simulink subsystem "PowerSystemRef"  (R2024b)
settings: Solver=VariableStepAuto  StartTime=0.0  StopTime=10.0  RelTol=1e-3
undefined symbols (not defined in the file): ess, geom, mot, mot2, mot3, mot4, propel, propel2, propel3, propel4, pxf_diagram_options, SimIn, tc, tc2, tc3, tc4
libraries: simulink x10, slpidlib x5
(part 8 of 10)

== system PowerSystemRef/powerplant/mot3/ctrl/dmd/parameter_selection ==
  inport-main_info_bus-1 : Inport
  select_main_info_bus : BusSelector  OutputSignals=apc_info_bus.apc_ctrl_dt3_simu,env_info_bus.env_plant_density_simu,apa_info_bus.powerplant_info_bus.ess.ctrl.ess_ctrl_pwr_max_pro_simu,apa_info_bus.powerplant_info_bus.propel3.propel3_plant_speed_simu,apa_info_bus.powerplant_info_bus.tc3.tc3_plant_spd_in_simu
  outport-apc_ctrl_dt3_simu-1 : Outport
  outport-env_plant_density_simu-2 : Outport  Port=2
  outport-ess_ctrl_pwr_max_pro_simu-3 : Outport  Port=3
  outport-propel3_plant_speed_simu-4 : Outport  Port=4
  outport-tc3_plant_spd_in_simu-5 : Outport  Port=5
  wires:
  inport-main_info_bus-1/1 -> select_main_info_bus/1
  select_main_info_bus/1 -> outport-apc_ctrl_dt3_simu-1/1  "<apc_ctrl_dt3_simu>"
  select_main_info_bus/2 -> outport-env_plant_density_simu-2/1  "<env_plant_density_simu>"
  select_main_info_bus/3 -> outport-ess_ctrl_pwr_max_pro_simu-3/1  "<ess_ctrl_pwr_max_pro_simu>"
  select_main_info_bus/4 -> outport-propel3_plant_speed_simu-4/1  "<propel3_plant_speed_simu>"
  select_main_info_bus/5 -> outport-tc3_plant_spd_in_simu-5/1  "<tc3_plant_spd_in_simu>"

== system PowerSystemRef/powerplant/mot3/plant/mot3_plant_map_Pelec_funTW_volt_in/electric machine filter ==
  trq : Inport
  Interval Test : simulink/Logic and Bit Operations/Interval Test  IntervalClosedRight=on  uplimit=0.02  IntervalClosedLeft=on  lowlimit=-0.02  OutDataTypeStr=boolean
  Switch : Switch  Threshold=0.5  SaturateOnIntegerOverflow=off  InputSameDT=off
  electric machine time response : TransferFcn  Denominator=[mot3.plant.init.time_response 1]
  filtered : Outport
  wires:
  Switch/1 -> filtered/1
  trq/1 -> electric machine time response/1, Interval Test/1, Switch/1
  Interval Test/1 -> Switch/2
  electric machine time response/1 -> Switch/3

== system PowerSystemRef/powerplant/mot3/plant/mot3_plant_map_Pelec_funTW_volt_in/max torque  ==
  cmd : Inport
  speed : Inport  Port=2
  torque : Inport  Port=3
  Abs : Abs
  Cont trq max - Prop : Subsystem  mask{x=mot3.plant.init.trq_pos_cont.idx1_spd, map=mot3.plant.init.trq_pos_cont.map}
      mask Display: image(imread('map1D.jpg','jpeg'))
  Cont trq max - Regen : Subsystem  mask{x=mot3.plant.init.trq_neg_cont.idx1_spd, map=mot3.plant.init.trq_neg_cont.map}
      mask Display: image(imread('map1D.jpg','jpeg'))
  Heat index : Subsystem
  Memory : Memory
  Peak trq max - Prop : Subsystem  mask{x=mot3.plant.init.trq_pos_max.idx1_spd, map=mot3.plant.init.trq_pos_max.map}
      mask Display: image(imread('map1D.jpg','jpeg'))
  Peak trq max - Regen : Subsystem  mask{x=mot3.plant.init.trq_neg_max.idx1_spd, map=mot3.plant.init.trq_neg_max.map}
      mask Display: image(imread('map1D.jpg','jpeg'))
  Product2 : Product  InputSameDT=on  SaturateOnIntegerOverflow=on  OutDataTypeStr=Inherit: Same as first input
  Product3 : Product  InputSameDT=on  SaturateOnIntegerOverflow=on  OutDataTypeStr=Inherit: Same as first input
  Product5 : Product  InputSameDT=on  SaturateOnIntegerOverflow=on  OutDataTypeStr=Inherit: Same as first input
  Sign : Signum
  Sum : Sum  InputSameDT=on  SaturateOnIntegerOverflow=on  OutDataTypeStr=Inherit: Same as first input
  Sum1 : Sum  Inputs=-+  InputSameDT=on  SaturateOnIntegerOverflow=on  OutDataTypeStr=Inherit: Same as first input
  Switch : Switch  InputSameDT=off
  Switch1 : Switch  InputSameDT=off
  cst : Constant
  max torque : Outport
  heat index : Outport  Port=2
  wires:
  Memory/1 -> Cont trq max - Prop/1(input x), Cont trq max - Regen/1(input x), Peak trq max - Regen/1(input x), Peak trq max - Prop/1(input x)
  Sign/1 -> Product5/1
  Product5/1 -> max torque/1
  Sum/1 -> Sign/1, Abs/1
  Abs/1 -> Product5/2
  torque/1 -> Heat index/2(torque)
  cmd/1 -> Switch1/2, Switch/2
  speed/1 -> Memory/1
  Cont trq max - Prop/1(output) -> Switch/1
  Cont trq max - Regen/1(output) -> Switch/3
  Peak trq max - Prop/1(output) -> Switch1/1
  Peak trq max - Regen/1(output) -> Switch1/3
  Switch/1 -> Product2/1, Heat index/1(cont torque)
  Switch1/1 -> Product3/2
  Product2/1 -> Sum/1
  Sum1/1 -> Product3/1
  Product3/1 -> Sum/2
  cst/1 -> Sum1/2
  Heat index/1(Heat index) -> Product2/2, Sum1/1, heat index/1

== system PowerSystemRef/powerplant/mot3/plant/mot3_plant_map_Pelec_funTW_volt_in/non-zero division ==
  note: and finally, the expression is: (u[1] \ u[2]) * 1 = u[1] \ u[2]
  note: (u[2]!=0) is true then returns 1
  note: if u[2] != 0, then output == u[1]\u[2]:
  note: (u[2]==0) is false then returns 0, thus (u[2]+(u[2]==0)) is equal to u[2]+0=u[2]
  note: and finally, the expression is: (u[1] \ 1) * 0 = 0
  note: (u[2]!=0) is false then returns 0
  note: if u[2] == 0, then output == 0:
  note: (u[2]==0) is true then returns 1, thus (u[2]+(u[2]==0)) is equal to 0+1=1
  note: original idea from Phil Sharer - ANL
      | original formula: u[1]\(u[2]+eps)*(u[2]!=0)
      | changes done by Gerald ZINI (dgey) - ANL (05\02\2001)
  In1 : Inport
  In2 : Inport  Port=2
  Fcn : Fcn  Expr=u[1]/(u[2]+(u[2]==0))*(u[2]!=0)
  Mux : Mux  Inputs=2
  Out1 : Outport
  wires:
  In2/1 -> Mux/2
  Fcn/1 -> Out1/1
  In1/1 -> Mux/1
  Mux/1 -> Fcn/1

== system PowerSystemRef/powerplant/mot4/ctrl/cmd/mot4_ctrl_cmd_map_Pelec_funTW_volt_in ==
  mot_plant_spd_out_simu : Inport
  mot_ctrl_trs_trq_simu : Inport  Port=2
  mot_ctrl_cstr_trq_max_pos_simu : Inport  Port=3
  mot_ctrl_cstr_trq_max_neg_simu : Inport  Port=4
  Abs : Abs
  Abs1 : Abs
  Abs2 : Abs
  Fcn : Fcn  Expr=(u>=0) - (u<0)
  Product : Product  SaturateOnIntegerOverflow=on  OutDataTypeStr=Inherit: Same as first input
  Product1 : Product  SaturateOnIntegerOverflow=on  OutDataTypeStr=Inherit: Same as first input
  Subsystem2 : Subsystem
      mask Display: disp('divider')
  Switch : Switch  InputSameDT=off
  "[-1, 1]" : Saturate  UpperLimit=1  LowerLimit=-1
  avoid zero output : Subsystem
  mot_ctrl_cmd_simu : Outport
  wires:
  avoid zero output/1(Out1) -> Product/2
  [mot4_ctrl_cmd_simu] -> mot_ctrl_cmd_simu/1  "mot_ctrl_cmd_simu"
  Product1/1 -> [mot4_ctrl_cmd_simu]
  mot_ctrl_cstr_trq_max_pos_simu/1 -> Abs1/1
  mot_ctrl_cstr_trq_max_neg_simu/1 -> Abs2/1
  mot_plant_spd_out_simu/1 -> avoid zero output/1(In1)
  Product/1 -> Switch/2, Fcn/1
  Switch/1 -> Subsystem2/2(In2)
  Subsystem2/1(Out1) -> "[-1, 1]"/1
  mot_ctrl_trs_trq_simu/1 -> Product/1, Abs/1
  Abs/1 -> Subsystem2/1(In1)
  Abs1/1 -> Switch/1
  Abs2/1 -> Switch/3
  "[-1, 1]"/1 -> Product1/2
  Fcn/1 -> Product1/1

== system PowerSystemRef/powerplant/mot4/ctrl/cmd/parameter_out ==
  inport-mot4_ctrl_cmd_simu : Inport
  Toworkspace-mot4_ctrl_cmd_simu : ToWorkspace  VariableName=mot4_ctrl_cmd_simu  SampleTime=pxf_diagram_options.workspace_sample_time
      settings: Decimation=pxf_diagram_options.decimation
  create_system_info_bus : BusCreator  Inputs=1
  outport-system_info_bus : Outport
  wires:
  create_system_info_bus/1 -> outport-system_info_bus/1
  inport-mot4_ctrl_cmd_simu/1 -> create_system_info_bus/1, Toworkspace-mot4_ctrl_cmd_simu/1  "mot4_ctrl_cmd_simu"

== system PowerSystemRef/powerplant/mot4/ctrl/cmd/parameter_selection ==
  inport-main_info_bus-1 : Inport
  select_main_info_bus : BusSelector  OutputSignals=apa_info_bus.powerplant_info_bus.mot4.plant.mot4_plant_spd_out_simu,apa_info_bus.powerplant_info_bus.mot4.ctrl.dmd.mot4_ctrl_trs_trq_simu,apa_info_bus.powerplant_info_bus.mot4.ctrl.cstr.mot4_ctrl_cstr_trq_max_pos_simu,apa_info_bus.powerplant_info_bus.mot4.ctrl.cstr.mot4_ctrl_cstr_trq_max_neg_simu
  outport-mot4_plant_spd_out_simu-1 : Outport
  outport-mot4_ctrl_trs_trq_simu-2 : Outport  Port=2
  outport-mot4_ctrl_cstr_trq_max_pos_simu-3 : Outport  Port=3
  outport-mot4_ctrl_cstr_trq_max_neg_simu-4 : Outport  Port=4
  wires:
  inport-main_info_bus-1/1 -> select_main_info_bus/1
  select_main_info_bus/1 -> outport-mot4_plant_spd_out_simu-1/1  "<mot4_plant_spd_out_simu>"
  select_main_info_bus/2 -> outport-mot4_ctrl_trs_trq_simu-2/1  "<mot4_ctrl_trs_trq_simu>"
  select_main_info_bus/3 -> outport-mot4_ctrl_cstr_trq_max_pos_simu-3/1  "<mot4_ctrl_cstr_trq_max_pos_simu>"
  select_main_info_bus/4 -> outport-mot4_ctrl_cstr_trq_max_neg_simu-4/1  "<mot4_ctrl_cstr_trq_max_neg_simu>"

== system PowerSystemRef/powerplant/mot4/ctrl/cstr/mot4_ctrl_cstr_map_Pelec_funTW_volt_in ==
  mot_plant_spd_out_simu : Inport
  mot_plant_temp_coeff_simu : Inport  Port=2
  Continuous torque - Prop : Subsystem  mask{x=mot4.plant.init.trq_pos_cont.idx1_spd, map=mot4.plant.init.trq_pos_cont.map}
      mask Display: image(imread('map1D.jpg','jpeg'))
  Continuous torque _regen : Subsystem  mask{x=mot4.plant.init.trq_neg_cont.idx1_spd, map=mot4.plant.init.trq_neg_cont.map}
      mask Display: image(imread('map1D.jpg','jpeg'))
  Mux1 : Mux  Inputs=3
  Mux2 : Mux  Inputs=3
  Peak torque - Prop : Subsystem  mask{x=mot4.plant.init.trq_pos_max.idx1_spd, map=mot4.plant.init.trq_pos_max.map}
      mask Display: image(imread('map1D.jpg','jpeg'))
  Peak torque _regen : Subsystem  mask{x=mot4.plant.init.trq_neg_max.idx1_spd, map=mot4.plant.init.trq_neg_max.map}
      mask Display: image(imread('map1D.jpg','jpeg'))
  Torque1 : Fcn  Expr=u[3]*(u[2] - u[1]) + u[1]
  max torque available from meca side : Fcn  Expr=u[3]*(u[2] - u[1]) + u[1]
  mot_ctrl_cstr_trq_pk_pos_simu : Outport
  mot_ctrl_cstr_trq_max_pos_simu : Outport  Port=2
  mot_ctrl_cstr_trq_pk_neg_simu : Outport  Port=3
  mot_ctrl_cstr_trq_max_neg_simu : Outport  Port=4
  mot_ctrl_cstr_trq_cont_pos_simu : Outport  Port=5
  mot_ctrl_cstr_trq_cont_neg_simu : Outport  Port=6
  mot_ctrl_cstr_temp_coeff_simu : Outport  Port=7
  wires:
  [mot4_ctrl_cstr_temp_coeff_simu] -> mot_ctrl_cstr_temp_coeff_simu/1  "mot_ctrl_cstr_temp_coeff_simu"
  [mot4_ctrl_cstr_trq_cont_neg_simu] -> mot_ctrl_cstr_trq_cont_neg_simu/1  "mot_ctrl_cstr_trq_cont_neg_simu"
  [mot4_ctrl_cstr_trq_cont_pos_simu] -> mot_ctrl_cstr_trq_cont_pos_simu/1  "mot_ctrl_cstr_trq_cont_pos_simu"
  [mot4_ctrl_cstr_trq_pk_neg_simu] -> mot_ctrl_cstr_trq_pk_neg_simu/1  "mot_ctrl_cstr_trq_pk_neg_simu"
  [mot4_ctrl_cstr_trq_max_neg_simu] -> mot_ctrl_cstr_trq_max_neg_simu/1  "mot_ctrl_cstr_trq_max_neg_simu"
  [mot4_ctrl_cstr_trq_max_pos_simu] -> mot_ctrl_cstr_trq_max_pos_simu/1  "mot_ctrl_cstr_trq_max_pos_simu"
  [mot4_ctrl_cstr_trq_pk_pos_simu] -> mot_ctrl_cstr_trq_pk_pos_simu/1  "mot_ctrl_cstr_trq_pk_pos_simu"
  mot_plant_spd_out_simu/1 -> Peak torque - Prop/1(input x), Continuous torque _regen/1(input x), Peak torque _regen/1(input x), Continuous torque - Prop/1(input x)
  Peak torque _regen/1(output) -> Mux1/1, [mot4_ctrl_cstr_trq_pk_neg_simu]
  Peak torque - Prop/1(output) -> [mot4_ctrl_cstr_trq_pk_pos_simu], Mux2/1
  mot_plant_temp_coeff_simu/1 -> [mot4_ctrl_cstr_temp_coeff_simu], Mux2/3, Mux1/3
  Mux1/1 -> Torque1/1
  Continuous torque _regen/1(output) -> [mot4_ctrl_cstr_trq_cont_neg_simu], Mux1/2
  Mux2/1 -> max torque available from meca side/1
  Continuous torque - Prop/1(output) -> [mot4_ctrl_cstr_trq_cont_pos_simu], Mux2/2
  Torque1/1 -> [mot4_ctrl_cstr_trq_max_neg_simu]
  max torque available from meca side/1 -> [mot4_ctrl_cstr_trq_max_pos_simu]

== system PowerSystemRef/powerplant/mot4/ctrl/cstr/parameter_out ==
  inport-mot4_ctrl_cstr_trq_pk_pos_simu : Inport
  inport-mot4_ctrl_cstr_trq_max_pos_simu : Inport  Port=2
  inport-mot4_ctrl_cstr_trq_pk_neg_simu : Inport  Port=3
  inport-mot4_ctrl_cstr_trq_max_neg_simu : Inport  Port=4
  inport-mot4_ctrl_cstr_trq_cont_pos_simu : Inport  Port=5
  inport-mot4_ctrl_cstr_trq_cont_neg_simu : Inport  Port=6
  inport-mot4_ctrl_cstr_temp_coeff_simu : Inport  Port=7
  Ground_1 : Ground
  Toworkspace-mot4_ctrl_cstr_temp_coeff_simu : ToWorkspace  VariableName=mot4_ctrl_cstr_temp_coeff_simu  SampleTime=pxf_diagram_options.workspace_sample_time
      settings: Decimation=pxf_diagram_options.decimation
  Toworkspace-mot4_ctrl_cstr_trq_cont_neg_simu : ToWorkspace  VariableName=mot4_ctrl_cstr_trq_cont_neg_simu  SampleTime=pxf_diagram_options.workspace_sample_time
      settings: Decimation=pxf_diagram_options.decimation
  Toworkspace-mot4_ctrl_cstr_trq_cont_pos_simu : ToWorkspace  VariableName=mot4_ctrl_cstr_trq_cont_pos_simu  SampleTime=pxf_diagram_options.workspace_sample_time
      settings: Decimation=pxf_diagram_options.decimation
  Toworkspace-mot4_ctrl_cstr_trq_max_neg_simu : ToWorkspace  VariableName=mot4_ctrl_cstr_trq_max_neg_simu  SampleTime=pxf_diagram_options.workspace_sample_time
      settings: Decimation=pxf_diagram_options.decimation
  Toworkspace-mot4_ctrl_cstr_trq_max_pos_simu : ToWorkspace  VariableName=mot4_ctrl_cstr_trq_max_pos_simu  SampleTime=pxf_diagram_options.workspace_sample_time
      settings: Decimation=pxf_diagram_options.decimation
  Toworkspace-mot4_ctrl_cstr_trq_pk_neg_simu : ToWorkspace  VariableName=mot4_ctrl_cstr_trq_pk_neg_simu  SampleTime=pxf_diagram_options.workspace_sample_time
      settings: Decimation=pxf_diagram_options.decimation
  Toworkspace-mot4_ctrl_cstr_trq_pk_pos_simu : ToWorkspace  VariableName=mot4_ctrl_cstr_trq_pk_pos_simu  SampleTime=pxf_diagram_options.workspace_sample_time
      settings: Decimation=pxf_diagram_options.decimation
  create_system_info_bus : BusCreator  Inputs=2
  outport-system_info_bus : Outport
  outport-cstr_bus : Outport  Port=2
  wires:
  create_system_info_bus/1 -> outport-system_info_bus/1
  inport-mot4_ctrl_cstr_trq_pk_pos_simu/1 -> Toworkspace-mot4_ctrl_cstr_trq_pk_pos_simu/1
  inport-mot4_ctrl_cstr_trq_max_pos_simu/1 -> create_system_info_bus/1, Toworkspace-mot4_ctrl_cstr_trq_max_pos_simu/1  "mot4_ctrl_cstr_trq_max_pos_simu"
  inport-mot4_ctrl_cstr_trq_pk_neg_simu/1 -> Toworkspace-mot4_ctrl_cstr_trq_pk_neg_simu/1
  inport-mot4_ctrl_cstr_trq_max_neg_simu/1 -> create_system_info_bus/2, Toworkspace-mot4_ctrl_cstr_trq_max_neg_simu/1  "mot4_ctrl_cstr_trq_max_neg_simu"
  inport-mot4_ctrl_cstr_trq_cont_pos_simu/1 -> Toworkspace-mot4_ctrl_cstr_trq_cont_pos_simu/1
  inport-mot4_ctrl_cstr_trq_cont_neg_simu/1 -> Toworkspace-mot4_ctrl_cstr_trq_cont_neg_simu/1
  inport-mot4_ctrl_cstr_temp_coeff_simu/1 -> Toworkspace-mot4_ctrl_cstr_temp_coeff_simu/1
  Ground_1/1 -> outport-cstr_bus/1

== system PowerSystemRef/powerplant/mot4/ctrl/cstr/parameter_selection ==
  inport-main_info_bus-1 : Inport
  select_main_info_bus : BusSelector  OutputSignals=apa_info_bus.powerplant_info_bus.mot4.plant.mot4_plant_spd_out_simu,apa_info_bus.powerplant_info_bus.mot4.plant.mot4_plant_temp_coeff_simu
  outport-mot4_plant_spd_out_simu-1 : Outport
  outport-mot4_plant_temp_coeff_simu-2 : Outport  Port=2
  wires:
  inport-main_info_bus-1/1 -> select_main_info_bus/1
  select_main_info_bus/1 -> outport-mot4_plant_spd_out_simu-1/1  "<mot4_plant_spd_out_simu>"
  select_main_info_bus/2 -> outport-mot4_plant_temp_coeff_simu-2/1  "<mot4_plant_temp_coeff_simu>"

== system PowerSystemRef/powerplant/mot4/ctrl/dmd/mot4_ctrl_dmd_uas ==
  apc_ctrl_dt_simu : Inport
  env_plant_density_simu : Inport  Port=2
  ess_ctrl_pwr_max_pro_simu : Inport  Port=3
  propel_plant_speed_simu : Inport  Port=4
  tc_plant_spd_in_simu : Inport  Port=5
  1\2pi1 : Gain  Gain=2*pi/mot4.tc.plant.init.ratio
  Constant : Constant  Value=mot4.propel.plant.init.Pmax
  Constant2 : Constant  Value=mot4.propel.init.CPpoly
  Constant3 : Constant  Value=0.01
  Constant8 : Constant  Value=mot4.propel.plant.init.propD
  Determine_Required_Motor_RPS : Subsystem
  Gain : Gain  Gain=1/2/pi
  Gain1 : Gain  Gain=1/2/pi
  PID Controller : slpidlib/PID Controller  Controller=PID  Form=Parallel  TimeDomain=Continuous-time  UseExternalTs=off  SampleTime=-1  IntegratorMethod=Forward Euler  FilterMethod=Forward Euler  ControllerParametersSource=internal  P=mot4.ctrl.init.P  I=mot4.ctrl.init.I  UseKiTs=off  D=mot4.ctrl.init.D  UseExternalDerivativeSource=off  N=100  UseFilter=on  TunerSelectOption=Transfer Function Based (PID Tuner App)  InitialConditionSource=internal  InitialConditionForIntegrator=0  InitialConditionForFilter=0  DifferentiatorICPrevScaledInput=0  ExternalReset=none  TrackingMode=off  Kt=1  LimitOutput=off  SatLimitsSource=internal  UpperSaturationLimit=inf  LowerSaturationLimit=-inf  LinearizeAsGain=on  AntiWindupMode=none  Kb=1  LimitIntegrator=off  UpperIntegratorSaturationLimit=inf  LowerIntegratorSaturationLimit=-inf  POutMin=[]  POutMax=[]  IOutMin=[]  IOutMax=[]  DOutMin=[]  DOutMax=[]  NOutMin=[]  NOutMax=[]  SumOutMin=[]  SumOutMax=[]  SaturationOutMin=[]  SaturationOutMax=[]  PParamMin=[]  PParamMax=[]  IParamMin=[]  IParamMax=[]  DParamMin=[]  DParamMax=[]  NParamMin=[]  NParamMax=[]  KbParamMin=[]  KbParamMax=[]  KtParamMin=[]  KtParamMax=[]  KbOutMin=[]  KbOutMax=[]  KtOutMin=[]  KtOutMax=[]  IntegratorOutMin=[]  IntegratorOutMax=[]  FilterOutMin=[]  FilterOutMax=[]  SumI1OutMin=[]  SumI1OutMax=[]  SumI2OutMin=[]  SumI2OutMax=[]  SumI3OutMin=[]  SumI3OutMax=[]  SumI4OutMin=[]  SumI4OutMax=[]  SumDOutMin=[]  SumDOutMax=[]  DifferentiatorOutMin=[]  DifferentiatorOutMax=[]  FilterDiffOutCoefMin=[]  FilterDiffOutCoefMax=[]  ReciprocalOutMin=[]  ReciprocalOutMax=[]  SumDenOutMin=[]  SumDenOutMax=[]  SumNumOutMin=[]  SumNumOutMax=[]  DivideOutMin=[]  DivideOutMax=[]  UdiffTsProdOutMin=[]  UdiffTsProdOutMax=[]  NTsProdOutMin=[]  NTsProdOutMax=[]  UintegralTsProdOutMin=[]  UintegralTsProdOutMax=[]  UngainTsProdOutMin=[]  UngainTsProdOutMax=[]  ClampingZeroOutDataTypeStr=Inherit: Inherit via back propagation  ClampingZeroOutMin=[]  ClampingZeroOutMax=[]  FilterDenConstantOutDataTypeStr=Inherit: Inherit via back propagation  FilterDenConstantOutMin=[]  FilterDenConstantOutMax=[]  PCopyOutDataTypeStr=Inherit: Inherit via back propagation  PCopyOutMin=[]  PCopyOutMax=[]  NCopyOutDataTypeStr=Inherit: Inherit via back propagation  NCopyOutMin=[]  NCopyOutMax=[]  IntegratorContinuousStateAttributes=''  IntegratorStateMustResolveToSignalObject=off  IntegratorRTWStateStorageClass=Auto  FilterContinuousStateAttributes=''  FilterStateMustResolveToSignalObject=off  FilterRTWStateStorageClass=Auto  ParallelPVariant=InternalParameters  IdealPVariant=Disabled  IVariant=InternalParameters  DVariant=InternalParameters  IntegratorVariant=Continuous  SatVariant=Disabled  AWVariant=Passthrough  PCopyVariant=Disabled  TRVariant=Disabled  FdbkBlocksVariant=Forward  IdealPFdbkVariant=Disabled  SatFdbkVariant=Disabled  DerivativeFilterVariant=ContFilter  NVariant=InternalParameters  NCopyVariant=Disabled  FilterICVariant=InternalICsFilter  IntegratorICVariant=InternalICs  ExternalResetVariant=Disabled  TRSumVariant=Passthrough  SumFdbkVariant=Disabled  SumVariant=Sum_PID  TsampFilterVariant=InternalTs  TsampNgainVariant=Passthrough  TsampIntegralVariant=Disabled_SignalSpec  ExternalSaturationOutDataTypeStr=Inherit: Same as second input  DerivativeSourceVariant=ErrorSignal  PreIntVariant=InternalPreInt
  Product2 : Product  RndMeth=Zero
  Product3 : Product
  Product4 : Product  Inputs=*/  RndMeth=Zero
  Saturation_Dynamic : simulink/Discontinuities/Saturation Dynamic  OutMin=[]  OutMax=[]  OutDataTypeStr=Inherit: Same as second input  OutDataType=fixdt(1, 16)  OutScaling=2^-10  DoSatur=off
  Sum2 : Sum  Inputs=+-|
  Sum3 : Sum  Inputs=|++
  mot_propel_plant_init_eff_map : Subsystem  mask{x=mot4.propel.plant.init.CP_CT_map(:,1)/60, map=mot4.propel.plant.init.CP_CT_map(:,4)}
  mot_ctrl_trs_trq_simu : Outport  VectorParamsAs1DForOutWhenUnconnected=off
  mot_ctrl_ratedpwr_simu : Outport  Port=2
  wires:
  Gain1/1 -> mot_propel_plant_init_eff_map/1(input x)
  Constant2/1 -> Determine_Required_Motor_RPS/4(CPpoly)
  env_plant_density_simu/1 -> Determine_Required_Motor_RPS/2(rho)
  Constant8/1 -> Determine_Required_Motor_RPS/1(Prop_D)
  Determine_Required_Motor_RPS/1(RPS_req) -> 1\2pi1/1, Sum2/1
  propel_plant_speed_simu/1 -> Gain1/1
  ess_ctrl_pwr_max_pro_simu/1 -> Saturation_Dynamic/1
  apc_ctrl_dt_simu/1 -> Product2/2
  Sum2/1 -> PID Controller/1
  1\2pi1/1 -> Product4/2
  Sum3/1 -> mot_ctrl_trs_trq_simu/1  "mot_ctrl_trs_trq_simu"
  PID Controller/1 -> Sum3/2
  Product4/1 -> Sum3/1  "required"
  Gain/1 -> Sum2/2  "actual"
  Product3/1 -> Saturation_Dynamic/2
  Saturation_Dynamic/1 -> Product4/1, Determine_Required_Motor_RPS/3(P)
  tc_plant_spd_in_simu/1 -> Gain/1
  Constant3/1 -> Saturation_Dynamic/3
  Constant/1 -> Product2/1, mot_ctrl_ratedpwr_simu/1  "mot_ctrl_ratedpwr_simu"
  mot_propel_plant_init_eff_map/1(output) -> Product3/2
  Product2/1 -> Product3/1

== system PowerSystemRef/powerplant/mot4/ctrl/dmd/parameter_out ==
  inport-mot4_ctrl_trs_trq_simu : Inport
  inport-mot4_ctrl_ratedpwr_simu : Inport  Port=2
  Ground_1 : Ground
  Toworkspace-mot4_ctrl_ratedpwr_simu : ToWorkspace  VariableName=mot4_ctrl_ratedpwr_simu  SampleTime=pxf_diagram_options.workspace_sample_time
      settings: Decimation=pxf_diagram_options.decimation
  Toworkspace-mot4_ctrl_trs_trq_simu : ToWorkspace  VariableName=mot4_ctrl_trs_trq_simu  SampleTime=pxf_diagram_options.workspace_sample_time
      settings: Decimation=pxf_diagram_options.decimation
  create_system_info_bus : BusCreator  Inputs=1
  outport-system_info_bus : Outport
  outport-dmd_bus : Outport  Port=2
  wires:
  create_system_info_bus/1 -> outport-system_info_bus/1
  inport-mot4_ctrl_trs_trq_simu/1 -> create_system_info_bus/1, Toworkspace-mot4_ctrl_trs_trq_simu/1  "mot4_ctrl_trs_trq_simu"
  inport-mot4_ctrl_ratedpwr_simu/1 -> Toworkspace-mot4_ctrl_ratedpwr_simu/1
  Ground_1/1 -> outport-dmd_bus/1

== system PowerSystemRef/powerplant/mot4/ctrl/dmd/parameter_selection ==
  inport-main_info_bus-1 : Inport
  select_main_info_bus : BusSelector  OutputSignals=apc_info_bus.apc_ctrl_dt4_simu,env_info_bus.env_plant_density_simu,apa_info_bus.powerplant_info_bus.ess.ctrl.ess_ctrl_pwr_max_pro_simu,apa_info_bus.powerplant_info_bus.propel4.propel4_plant_speed_simu,apa_info_bus.powerplant_info_bus.tc4.tc4_plant_spd_in_simu
  outport-apc_ctrl_dt4_simu-1 : Outport
  outport-env_plant_density_simu-2 : Outport  Port=2
  outport-ess_ctrl_pwr_max_pro_simu-3 : Outport  Port=3
  outport-propel4_plant_speed_simu-4 : Outport  Port=4
  outport-tc4_plant_spd_in_simu-5 : Outport  Port=5
  wires:
  inport-main_info_bus-1/1 -> select_main_info_bus/1
  select_main_info_bus/1 -> outport-apc_ctrl_dt4_simu-1/1  "<apc_ctrl_dt4_simu>"
  select_main_info_bus/2 -> outport-env_plant_density_simu-2/1  "<env_plant_density_simu>"
  select_main_info_bus/3 -> outport-ess_ctrl_pwr_max_pro_simu-3/1  "<ess_ctrl_pwr_max_pro_simu>"
  select_main_info_bus/4 -> outport-propel4_plant_speed_simu-4/1  "<propel4_plant_speed_simu>"
  select_main_info_bus/5 -> outport-tc4_plant_spd_in_simu-5/1  "<tc4_plant_spd_in_simu>"

== system PowerSystemRef/powerplant/mot4/plant/mot4_plant_map_Pelec_funTW_volt_in/electric machine filter ==
  trq : Inport
  Interval Test : simulink/Logic and Bit Operations/Interval Test  IntervalClosedRight=on  uplimit=0.02  IntervalClosedLeft=on  lowlimit=-0.02  OutDataTypeStr=boolean
  Switch : Switch  Threshold=0.5  SaturateOnIntegerOverflow=off  InputSameDT=off
  electric machine time response : TransferFcn  Denominator=[mot4.plant.init.time_response 1]
  filtered : Outport
  wires:
  Switch/1 -> filtered/1
  trq/1 -> electric machine time response/1, Interval Test/1, Switch/1
  Interval Test/1 -> Switch/2
  electric machine time response/1 -> Switch/3

== system PowerSystemRef/powerplant/mot4/plant/mot4_plant_map_Pelec_funTW_volt_in/max torque  ==
  cmd : Inport
  speed : Inport  Port=2
  torque : Inport  Port=3
  Abs : Abs
  Cont trq max - Prop : Subsystem  mask{x=mot4.plant.init.trq_pos_cont.idx1_spd, map=mot4.plant.init.trq_pos_cont.map}
      mask Display: image(imread('map1D.jpg','jpeg'))
  Cont trq max - Regen : Subsystem  mask{x=mot4.plant.init.trq_neg_cont.idx1_spd, map=mot4.plant.init.trq_neg_cont.map}
      mask Display: image(imread('map1D.jpg','jpeg'))
  Heat index : Subsystem
  Memory : Memory
  Peak trq max - Prop : Subsystem  mask{x=mot4.plant.init.trq_pos_max.idx1_spd, map=mot4.plant.init.trq_pos_max.map}
      mask Display: image(imread('map1D.jpg','jpeg'))
  Peak trq max - Regen : Subsystem  mask{x=mot4.plant.init.trq_neg_max.idx1_spd, map=mot4.plant.init.trq_neg_max.map}
      mask Display: image(imread('map1D.jpg','jpeg'))
  Product2 : Product  InputSameDT=on  SaturateOnIntegerOverflow=on  OutDataTypeStr=Inherit: Same as first input
  Product3 : Product  InputSameDT=on  SaturateOnIntegerOverflow=on  OutDataTypeStr=Inherit: Same as first input
  Product5 : Product  InputSameDT=on  SaturateOnIntegerOverflow=on  OutDataTypeStr=Inherit: Same as first input
  Sign : Signum
  Sum : Sum  InputSameDT=on  SaturateOnIntegerOverflow=on  OutDataTypeStr=Inherit: Same as first input
  Sum1 : Sum  Inputs=-+  InputSameDT=on  SaturateOnIntegerOverflow=on  OutDataTypeStr=Inherit: Same as first input
  Switch : Switch  InputSameDT=off
  Switch1 : Switch  InputSameDT=off
  cst : Constant
  max torque : Outport
  heat index : Outport  Port=2
  wires:
  Memory/1 -> Cont trq max - Prop/1(input x), Cont trq max - Regen/1(input x), Peak trq max - Regen/1(input x), Peak trq max - Prop/1(input x)
  Sign/1 -> Product5/1
  Product5/1 -> max torque/1
  Sum/1 -> Sign/1, Abs/1
  Abs/1 -> Product5/2
  torque/1 -> Heat index/2(torque)
  cmd/1 -> Switch1/2, Switch/2
  speed/1 -> Memory/1
  Cont trq max - Prop/1(output) -> Switch/1
  Cont trq max - Regen/1(output) -> Switch/3
  Peak trq max - Prop/1(output) -> Switch1/1
  Peak trq max - Regen/1(output) -> Switch1/3
  Switch/1 -> Product2/1, Heat index/1(cont torque)
  Switch1/1 -> Product3/2
  Product2/1 -> Sum/1
  Sum1/1 -> Product3/1
  Product3/1 -> Sum/2
  cst/1 -> Sum1/2
  Heat index/1(Heat index) -> Product2/2, Sum1/1, heat index/1

== system PowerSystemRef/powerplant/mot4/plant/mot4_plant_map_Pelec_funTW_volt_in/non-zero division ==
  note: and finally, the expression is: (u[1] \ u[2]) * 1 = u[1] \ u[2]
  note: (u[2]!=0) is true then returns 1
  note: if u[2] != 0, then output == u[1]\u[2]:
  note: (u[2]==0) is false then returns 0, thus (u[2]+(u[2]==0)) is equal to u[2]+0=u[2]
  note: and finally, the expression is: (u[1] \ 1) * 0 = 0
  note: (u[2]!=0) is false then returns 0
  note: if u[2] == 0, then output == 0:
  note: (u[2]==0) is true then returns 1, thus (u[2]+(u[2]==0)) is equal to 0+1=1
  note: original idea from Phil Sharer - ANL
      | original formula: u[1]\(u[2]+eps)*(u[2]!=0)
      | changes done by Gerald ZINI (dgey) - ANL (05\02\2001)
  In1 : Inport
  In2 : Inport  Port=2
  Fcn : Fcn  Expr=u[1]/(u[2]+(u[2]==0))*(u[2]!=0)
  Mux : Mux  Inputs=2
  Out1 : Outport
  wires:
  In2/1 -> Mux/2
  Fcn/1 -> Out1/1
  In1/1 -> Mux/1
  Mux/1 -> Fcn/1

== system PowerSystemRef/powerplant/propel/plant/propel_plant_uas/Propeller Power ==
  propel_plant_CT_simu : Inport
  propel_plant_CP_simu : Inport  Port=2
  propel_plant_thrust_simu : Inport  Port=3
  propel_plant_rps_simu : Inport  Port=4
  eqnmotion_plant_linvel_simu : Inport  Port=5
  Dot Product : DotProduct  OutDataTypeStr=Inherit: Inherit via internal rule
  Fcn : Fcn  Expr=u(2) / u(1) * u(4) * u(3) * propel.plant.init.propD
  Mux : Mux
  Product : Product
  Sqrt : Sqrt
  propel_plant_pwr_in_simu : Outport  VectorParamsAs1DForOutWhenUnconnected=off
  propel_plant_pwr_out_simu : Outport  Port=2  VectorParamsAs1DForOutWhenUnconnected=off
  wires:
  Dot Product/1 -> Sqrt/1
  eqnmotion_plant_linvel_simu/1 -> Dot Product/1, Dot Product/2
  Sqrt/1 -> Product/2  "tas"
  Product/1 -> propel_plant_pwr_out_simu/1
  Mux/1 -> Fcn/1
  propel_plant_CT_simu/1 -> Mux/1
  propel_plant_thrust_simu/1 -> Mux/3, Product/1
  propel_plant_rps_simu/1 -> Mux/4
  Fcn/1 -> propel_plant_pwr_in_simu/1  "propel_plant_pwr_in_simu"
  propel_plant_CP_simu/1 -> Mux/2

== system PowerSystemRef/powerplant/propel/plant/propel_plant_uas/Propeller_CP ==
  propel_plant_rps_simu : Inport
  propel_plant_init_CP_CT_map : Subsystem  mask{x=propel.plant.init.CP_CT_map(:,1)/60, map=propel.plant.init.CP_CT_map(:,3)}
  propel_plant_CP_simu : Outport  VectorParamsAs1DForOutWhenUnconnected=off
  wires:
  propel_plant_init_CP_CT_map/1(output) -> propel_plant_CP_simu/1
  propel_plant_rps_simu/1 -> propel_plant_init_CP_CT_map/1(input x)

== system PowerSystemRef/powerplant/propel/plant/propel_plant_uas/Propeller_Torque ==
  note: I = Wprop*R^2/3g
      | General Aviation Aircraft Design pg 619
  env_plant_density_simu : Inport
  propel_plant_CP_simu : Inport  Port=2
  tc_plant_trq_out_simu : Inport  Port=3
  tc_plant_inertia_out_simu : Inport  Port=4
  " " : Gain  Gain=-1
  "2pi " : Gain  Gain=1/2/pi
  Demux : Demux  Outputs=2
  Fcn1 : Fcn  Expr=(u(1)/(2*pi)) *u(3)*(u(2)^2)*(propel.plant.init.propD^5)
  Integrator1 : Integrator  InitialCondition=propel.ctrl.init.rps
  Mux : Mux  Inputs=3
  Product : Product  Inputs=*/
  Prop Inertia : Constant  Value=propel.plant.init.Iprop
  Sum1 : Sum  Inputs=|+-
  Sum2 : Sum  Inputs=|++
  Terminator : Terminator
  propel_plant_rps_simu : Outport  VectorParamsAs1DForOutWhenUnconnected=off
  propel_plant_restq_simu : Outport  Port=2  VectorParamsAs1DForOutWhenUnconnected=off
  wires:
  Demux/2 -> Terminator/1
  Demux/1 -> Sum1/1
  "2pi "/1 -> Integrator1/1
  Mux/1 -> Fcn1/1
  " "/1 -> propel_plant_restq_simu/1
  Integrator1/1 -> propel_plant_rps_simu/1, Mux/2  "propeller_plant_rps_simu"
  env_plant_density_simu/1 -> Mux/3  "env_plant_density_simu"
  propel_plant_CP_simu/1 -> Mux/1  "prop_plant_CP_simu"
  tc_plant_trq_out_simu/1 -> Demux/1
  Fcn1/1 -> Sum1/2, " "/1  "propel_plant_restq_simu"
  Prop Inertia/1 -> Sum2/1
  tc_plant_inertia_out_simu/1 -> Sum2/2
  Sum2/1 -> Product/2
  Sum1/1 -> Product/1
  Product/1 -> "2pi "/1

== system PowerSystemRef/powerplant/propel/plant/propel_plant_uas/Thrust_Generated ==
  env_plant_density_simu : Inport
  propel_plant_speed_simu : Inport  Port=2
  Mux5 : Mux  Inputs=3
  RPS2T : Fcn  Expr=u(2) * u(3) * propel.plant.init.propD^4 * u(1)^2
  propel_plant_init_CP_CT_map : Subsystem  mask{x=propel.plant.init.CP_CT_map(:,1)/60, map=propel.plant.init.CP_CT_map(:,2)}
  propel_plant_thrust_simu : Outport  VectorParamsAs1DForOutWhenUnconnected=off
  propel_plant_CT_simu : Outport  Port=2  VectorParamsAs1DForOutWhenUnconnected=off
  wires:
  propel_plant_init_CP_CT_map/1(output) -> propel_plant_CT_simu/1, Mux5/2
  env_plant_density_simu/1 -> Mux5/3
  propel_plant_speed_simu/1 -> propel_plant_init_CP_CT_map/1(input x), Mux5/1
  Mux5/1 -> RPS2T/1
  RPS2T/1 -> propel_plant_thrust_simu/1

== system PowerSystemRef/powerplant/propel/plant/propel_plant_uas/Total_Moment ==
  propel_plant_thrust_simu : Inport
  propel_plant_restq_simu : Inport  Port=2
  Gain : Gain  Gain=-propel.plant.init.rotationdir
  Gain1 : Gain  Gain=propel.plant.init.thrustdir
  Moment_due_to_eng_position : Subsystem
  Sum2 : Sum  Inputs=|+-  SaturateOnIntegerOverflow=on
  Sum4 : Sum  SaturateOnIntegerOverflow=on
  geom.init.CG : Constant  Value=geom.init.CG
  propel.plant.init.pos : Constant  Value=propel.plant.init.pos
  accmoment_plant_totmoment_simu : Outport  VectorParamsAs1DForOutWhenUnconnected=off
  wires:
  propel_plant_restq_simu/1 -> Gain/1
  Gain1/1 -> Moment_due_to_eng_position/2(Vec 2)
  Gain/1 -> Sum4/2
  Sum2/1 -> Moment_due_to_eng_position/1(Vec 1)
  Sum4/1 -> accmoment_plant_totmoment_simu/1  "accmoment_plant_totmoment_simu"
  propel.plant.init.pos/1 -> Sum2/1
  geom.init.CG/1 -> Sum2/2
  propel_plant_thrust_simu/1 -> Gain1/1
  Moment_due_to_eng_position/1(X Prod) -> Sum4/1

== system PowerSystemRef/powerplant/propel2/plant/propel2_plant_uas/Propeller Power ==
  propel_plant_CT_simu : Inport
  propel_plant_CP_simu : Inport  Port=2
  propel_plant_thrust_simu : Inport  Port=3
  propel_plant_rps_simu : Inport  Port=4
  eqnmotion_plant_linvel_simu : Inport  Port=5
  Dot Product : DotProduct  OutDataTypeStr=Inherit: Inherit via internal rule
  Fcn : Fcn  Expr=u(2) / u(1) * u(4) * u(3) * propel2.plant.init.propD
  Mux : Mux
  Product : Product
  Sqrt : Sqrt
  propel_plant_pwr_in_simu : Outport  VectorParamsAs1DForOutWhenUnconnected=off
  propel_plant_pwr_out_simu : Outport  Port=2  VectorParamsAs1DForOutWhenUnconnected=off
  wires:
  Dot Product/1 -> Sqrt/1
  eqnmotion_plant_linvel_simu/1 -> Dot Product/1, Dot Product/2
  Sqrt/1 -> Product/2  "tas"
  Product/1 -> propel_plant_pwr_out_simu/1
  Mux/1 -> Fcn/1
  propel_plant_CT_simu/1 -> Mux/1
  propel_plant_thrust_simu/1 -> Mux/3, Product/1
  propel_plant_rps_simu/1 -> Mux/4
  Fcn/1 -> propel_plant_pwr_in_simu/1  "propel_plant_pwr_in_simu"
  propel_plant_CP_simu/1 -> Mux/2

== system PowerSystemRef/powerplant/propel2/plant/propel2_plant_uas/Propeller_CP ==
  propel_plant_rps_simu : Inport
  propel_plant_init_CP_CT_map : Subsystem  mask{x=propel2.plant.init.CP_CT_map(:,1)/60, map=propel2.plant.init.CP_CT_map(:,3)}
  propel_plant_CP_simu : Outport  VectorParamsAs1DForOutWhenUnconnected=off
  wires:
  propel_plant_init_CP_CT_map/1(output) -> propel_plant_CP_simu/1
  propel_plant_rps_simu/1 -> propel_plant_init_CP_CT_map/1(input x)

== system PowerSystemRef/powerplant/propel2/plant/propel2_plant_uas/Propeller_Torque ==
  note: I = Wprop*R^2/3g
      | General Aviation Aircraft Design pg 619
  env_plant_density_simu : Inport
  propel_plant_CP_simu : Inport  Port=2
  tc_plant_trq_out_simu : Inport  Port=3
  tc_plant_inertia_out_simu : Inport  Port=4
  " " : Gain  Gain=-1
  "2pi " : Gain  Gain=1/2/pi
  Demux : Demux  Outputs=2
  Fcn1 : Fcn  Expr=(u(1)/(2*pi)) *u(3)*(u(2)^2)*(propel2.plant.init.propD^5)
  Integrator1 : Integrator  InitialCondition=propel2.ctrl.init.rps
  Mux : Mux  Inputs=3
  Product : Product  Inputs=*/
  Prop Inertia : Constant  Value=propel2.plant.init.Iprop
  Sum1 : Sum  Inputs=|+-
  Sum2 : Sum  Inputs=|++
  Terminator : Terminator
  propel_plant_rps_simu : Outport  VectorParamsAs1DForOutWhenUnconnected=off
  propel_plant_restq_simu : Outport  Port=2  VectorParamsAs1DForOutWhenUnconnected=off
  wires:
  Demux/2 -> Terminator/1
  Demux/1 -> Sum1/1
  "2pi "/1 -> Integrator1/1
  Mux/1 -> Fcn1/1
  " "/1 -> propel_plant_restq_simu/1
  Integrator1/1 -> propel_plant_rps_simu/1, Mux/2  "propeller_plant_rps_simu"
  env_plant_density_simu/1 -> Mux/3  "env_plant_density_simu"
  propel_plant_CP_simu/1 -> Mux/1  "prop_plant_CP_simu"
  tc_plant_trq_out_simu/1 -> Demux/1
  Fcn1/1 -> Sum1/2, " "/1  "propel_plant_restq_simu"
  Prop Inertia/1 -> Sum2/1
  tc_plant_inertia_out_simu/1 -> Sum2/2
  Sum2/1 -> Product/2
  Sum1/1 -> Product/1
  Product/1 -> "2pi "/1

== system PowerSystemRef/powerplant/propel2/plant/propel2_plant_uas/Thrust_Generated ==
  env_plant_density_simu : Inport
  propel_plant_speed_simu : Inport  Port=2
  Mux5 : Mux  Inputs=3
  RPS2T : Fcn  Expr=u(2) * u(3) * propel2.plant.init.propD^4 * u(1)^2
  propel_plant_init_CP_CT_map : Subsystem  mask{x=propel2.plant.init.CP_CT_map(:,1)/60, map=propel2.plant.init.CP_CT_map(:,2)}
  propel_plant_thrust_simu : Outport  VectorParamsAs1DForOutWhenUnconnected=off
  propel_plant_CT_simu : Outport  Port=2  VectorParamsAs1DForOutWhenUnconnected=off
  wires:
  propel_plant_init_CP_CT_map/1(output) -> propel_plant_CT_simu/1, Mux5/2
  env_plant_density_simu/1 -> Mux5/3
  propel_plant_speed_simu/1 -> propel_plant_init_CP_CT_map/1(input x), Mux5/1
  Mux5/1 -> RPS2T/1
  RPS2T/1 -> propel_plant_thrust_simu/1

== system PowerSystemRef/powerplant/propel2/plant/propel2_plant_uas/Total_Moment ==
  propel_plant_thrust_simu : Inport
  propel_plant_restq_simu : Inport  Port=2
  Gain : Gain  Gain=-propel2.plant.init.rotationdir
  Gain1 : Gain  Gain=propel2.plant.init.thrustdir
  Moment_due_to_eng_position : Subsystem
  Sum2 : Sum  Inputs=|+-  SaturateOnIntegerOverflow=on
  Sum4 : Sum  SaturateOnIntegerOverflow=on
  geom.init.CG : Constant  Value=geom.init.CG
  propel.plant.init.pos : Constant  Value=propel2.plant.init.pos
  accmoment_plant_totmoment_simu : Outport  VectorParamsAs1DForOutWhenUnconnected=off
  wires:
  propel_plant_restq_simu/1 -> Gain/1
  Gain1/1 -> Moment_due_to_eng_position/2(Vec 2)
  Gain/1 -> Sum4/2
  Sum2/1 -> Moment_due_to_eng_position/1(Vec 1)
  Sum4/1 -> accmoment_plant_totmoment_simu/1  "accmoment_plant_totmoment_simu"
  propel.plant.init.pos/1 -> Sum2/1
  geom.init.CG/1 -> Sum2/2
  propel_plant_thrust_simu/1 -> Gain1/1
  Moment_due_to_eng_position/1(X Prod) -> Sum4/1

== system PowerSystemRef/powerplant/propel3/plant/propel3_plant_uas/Propeller Power ==
  propel_plant_CT_simu : Inport
  propel_plant_CP_simu : Inport  Port=2
  propel_plant_thrust_simu : Inport  Port=3
  propel_plant_rps_simu : Inport  Port=4
  eqnmotion_plant_linvel_simu : Inport  Port=5
  Dot Product : DotProduct  OutDataTypeStr=Inherit: Inherit via internal rule
  Fcn : Fcn  Expr=u(2) / u(1) * u(4) * u(3) * propel3.plant.init.propD
  Mux : Mux
  Product : Product
  Sqrt : Sqrt
  propel_plant_pwr_in_simu : Outport  VectorParamsAs1DForOutWhenUnconnected=off
  propel_plant_pwr_out_simu : Outport  Port=2  VectorParamsAs1DForOutWhenUnconnected=off
  wires:
  Dot Product/1 -> Sqrt/1
  eqnmotion_plant_linvel_simu/1 -> Dot Product/1, Dot Product/2
  Sqrt/1 -> Product/2  "tas"
  Product/1 -> propel_plant_pwr_out_simu/1
  Mux/1 -> Fcn/1
  propel_plant_CT_simu/1 -> Mux/1
  propel_plant_thrust_simu/1 -> Mux/3, Product/1
  propel_plant_rps_simu/1 -> Mux/4
  Fcn/1 -> propel_plant_pwr_in_simu/1  "propel_plant_pwr_in_simu"
  propel_plant_CP_simu/1 -> Mux/2

== system PowerSystemRef/powerplant/propel3/plant/propel3_plant_uas/Propeller_CP ==
  propel_plant_rps_simu : Inport
  propel_plant_init_CP_CT_map : Subsystem  mask{x=propel3.plant.init.CP_CT_map(:,1)/60, map=propel3.plant.init.CP_CT_map(:,3)}
  propel_plant_CP_simu : Outport  VectorParamsAs1DForOutWhenUnconnected=off
  wires:
  propel_plant_init_CP_CT_map/1(output) -> propel_plant_CP_simu/1
  propel_plant_rps_simu/1 -> propel_plant_init_CP_CT_map/1(input x)

== system PowerSystemRef/powerplant/propel3/plant/propel3_plant_uas/Propeller_Torque ==
  note: I = Wprop*R^2/3g
      | General Aviation Aircraft Design pg 619
  env_plant_density_simu : Inport
  propel_plant_CP_simu : Inport  Port=2
  tc_plant_trq_out_simu : Inport  Port=3
  tc_plant_inertia_out_simu : Inport  Port=4
  " " : Gain  Gain=-1
  "2pi " : Gain  Gain=1/2/pi
  Demux : Demux  Outputs=2
  Fcn1 : Fcn  Expr=(u(1)/(2*pi)) *u(3)*(u(2)^2)*(propel3.plant.init.propD^5)
  Integrator1 : Integrator  InitialCondition=propel3.ctrl.init.rps
  Mux : Mux  Inputs=3
  Product : Product  Inputs=*/
  Prop Inertia : Constant  Value=propel3.plant.init.Iprop
  Sum1 : Sum  Inputs=|+-
  Sum2 : Sum  Inputs=|++
  Terminator : Terminator
  propel_plant_rps_simu : Outport  VectorParamsAs1DForOutWhenUnconnected=off
  propel_plant_restq_simu : Outport  Port=2  VectorParamsAs1DForOutWhenUnconnected=off
  wires:
  Demux/2 -> Terminator/1
  Demux/1 -> Sum1/1
  "2pi "/1 -> Integrator1/1
  Mux/1 -> Fcn1/1
  " "/1 -> propel_plant_restq_simu/1
  Integrator1/1 -> propel_plant_rps_simu/1, Mux/2  "propeller_plant_rps_simu"
  env_plant_density_simu/1 -> Mux/3  "env_plant_density_simu"
  propel_plant_CP_simu/1 -> Mux/1  "prop_plant_CP_simu"
  tc_plant_trq_out_simu/1 -> Demux/1
  Fcn1/1 -> Sum1/2, " "/1  "propel_plant_restq_simu"
  Prop Inertia/1 -> Sum2/1
  tc_plant_inertia_out_simu/1 -> Sum2/2
  Sum2/1 -> Product/2
  Sum1/1 -> Product/1
  Product/1 -> "2pi "/1

== system PowerSystemRef/powerplant/propel3/plant/propel3_plant_uas/Thrust_Generated ==
  env_plant_density_simu : Inport
  propel_plant_speed_simu : Inport  Port=2
  Mux5 : Mux  Inputs=3
  RPS2T : Fcn  Expr=u(2) * u(3) * propel3.plant.init.propD^4 * u(1)^2
  propel_plant_init_CP_CT_map : Subsystem  mask{x=propel3.plant.init.CP_CT_map(:,1)/60, map=propel3.plant.init.CP_CT_map(:,2)}
  propel_plant_thrust_simu : Outport  VectorParamsAs1DForOutWhenUnconnected=off
  propel_plant_CT_simu : Outport  Port=2  VectorParamsAs1DForOutWhenUnconnected=off
  wires:
  propel_plant_init_CP_CT_map/1(output) -> propel_plant_CT_simu/1, Mux5/2
  env_plant_density_simu/1 -> Mux5/3
  propel_plant_speed_simu/1 -> propel_plant_init_CP_CT_map/1(input x), Mux5/1
  Mux5/1 -> RPS2T/1
  RPS2T/1 -> propel_plant_thrust_simu/1

== system PowerSystemRef/powerplant/propel3/plant/propel3_plant_uas/Total_Moment ==
  propel_plant_thrust_simu : Inport
  propel_plant_restq_simu : Inport  Port=2
  Gain : Gain  Gain=-propel3.plant.init.rotationdir
  Gain1 : Gain  Gain=propel3.plant.init.thrustdir
  Moment_due_to_eng_position : Subsystem
  Sum2 : Sum  Inputs=|+-  SaturateOnIntegerOverflow=on
  Sum4 : Sum  SaturateOnIntegerOverflow=on
  geom.init.CG : Constant  Value=geom.init.CG
  propel.plant.init.pos : Constant  Value=propel3.plant.init.pos
  accmoment_plant_totmoment_simu : Outport  VectorParamsAs1DForOutWhenUnconnected=off
  wires:
  propel_plant_restq_simu/1 -> Gain/1
  Gain1/1 -> Moment_due_to_eng_position/2(Vec 2)
  Gain/1 -> Sum4/2
  Sum2/1 -> Moment_due_to_eng_position/1(Vec 1)
  Sum4/1 -> accmoment_plant_totmoment_simu/1  "accmoment_plant_totmoment_simu"
  propel.plant.init.pos/1 -> Sum2/1
  geom.init.CG/1 -> Sum2/2
  propel_plant_thrust_simu/1 -> Gain1/1
  Moment_due_to_eng_position/1(X Prod) -> Sum4/1

== system PowerSystemRef/powerplant/propel4/plant/propel4_plant_uas/Propeller Power ==
  propel_plant_CT_simu : Inport
  propel_plant_CP_simu : Inport  Port=2
  propel_plant_thrust_simu : Inport  Port=3
  propel_plant_rps_simu : Inport  Port=4
  eqnmotion_plant_linvel_simu : Inport  Port=5
  Dot Product : DotProduct  OutDataTypeStr=Inherit: Inherit via internal rule
  Fcn : Fcn  Expr=u(2) / u(1) * u(4) * u(3) * propel4.plant.init.propD
  Mux : Mux
  Product : Product
  Sqrt : Sqrt
  propel_plant_pwr_in_simu : Outport  VectorParamsAs1DForOutWhenUnconnected=off
  propel_plant_pwr_out_simu : Outport  Port=2  VectorParamsAs1DForOutWhenUnconnected=off
  wires:
  Dot Product/1 -> Sqrt/1
  eqnmotion_plant_linvel_simu/1 -> Dot Product/1, Dot Product/2
  Sqrt/1 -> Product/2  "tas"
  Product/1 -> propel_plant_pwr_out_simu/1
  Mux/1 -> Fcn/1
  propel_plant_CT_simu/1 -> Mux/1
  propel_plant_thrust_simu/1 -> Mux/3, Product/1
  propel_plant_rps_simu/1 -> Mux/4
  Fcn/1 -> propel_plant_pwr_in_simu/1  "propel_plant_pwr_in_simu"
  propel_plant_CP_simu/1 -> Mux/2

== system PowerSystemRef/powerplant/propel4/plant/propel4_plant_uas/Propeller_CP ==
  propel_plant_rps_simu : Inport
  propel_plant_init_CP_CT_map : Subsystem  mask{x=propel4.plant.init.CP_CT_map(:,1)/60, map=propel4.plant.init.CP_CT_map(:,3)}
  propel_plant_CP_simu : Outport  VectorParamsAs1DForOutWhenUnconnected=off
  wires:
  propel_plant_init_CP_CT_map/1(output) -> propel_plant_CP_simu/1
  propel_plant_rps_simu/1 -> propel_plant_init_CP_CT_map/1(input x)

== system PowerSystemRef/powerplant/propel4/plant/propel4_plant_uas/Propeller_Torque ==
  note: I = Wprop*R^2/3g
      | General Aviation Aircraft Design pg 619
  env_plant_density_simu : Inport
  propel_plant_CP_simu : Inport  Port=2
  tc_plant_trq_out_simu : Inport  Port=3
  tc_plant_inertia_out_simu : Inport  Port=4
  " " : Gain  Gain=-1
  "2pi " : Gain  Gain=1/2/pi
  Demux : Demux  Outputs=2
  Fcn1 : Fcn  Expr=(u(1)/(2*pi)) *u(3)*(u(2)^2)*(propel4.plant.init.propD^5)
  Integrator1 : Integrator  InitialCondition=propel4.ctrl.init.rps
  Mux : Mux  Inputs=3
  Product : Product  Inputs=*/
  Prop Inertia : Constant  Value=propel4.plant.init.Iprop
  Sum1 : Sum  Inputs=|+-
  Sum2 : Sum  Inputs=|++
  Terminator : Terminator
  propel_plant_rps_simu : Outport  VectorParamsAs1DForOutWhenUnconnected=off
  propel_plant_restq_simu : Outport  Port=2  VectorParamsAs1DForOutWhenUnconnected=off
  wires:
  Demux/2 -> Terminator/1
  Demux/1 -> Sum1/1
  "2pi "/1 -> Integrator1/1
  Mux/1 -> Fcn1/1
  " "/1 -> propel_plant_restq_simu/1
  Integrator1/1 -> propel_plant_rps_simu/1, Mux/2  "propeller_plant_rps_simu"
  env_plant_density_simu/1 -> Mux/3  "env_plant_density_simu"
  propel_plant_CP_simu/1 -> Mux/1  "prop_plant_CP_simu"
  tc_plant_trq_out_simu/1 -> Demux/1
  Fcn1/1 -> Sum1/2, " "/1  "propel_plant_restq_simu"
  Prop Inertia/1 -> Sum2/1
  tc_plant_inertia_out_simu/1 -> Sum2/2
  Sum2/1 -> Product/2
  Sum1/1 -> Product/1
  Product/1 -> "2pi "/1

== system PowerSystemRef/powerplant/propel4/plant/propel4_plant_uas/Thrust_Generated ==
  env_plant_density_simu : Inport
  propel_plant_speed_simu : Inport  Port=2
  Mux5 : Mux  Inputs=3
  RPS2T : Fcn  Expr=u(2) * u(3) * propel4.plant.init.propD^4 * u(1)^2
  propel_plant_init_CP_CT_map : Subsystem  mask{x=propel4.plant.init.CP_CT_map(:,1)/60, map=propel4.plant.init.CP_CT_map(:,2)}
  propel_plant_thrust_simu : Outport  VectorParamsAs1DForOutWhenUnconnected=off
  propel_plant_CT_simu : Outport  Port=2  VectorParamsAs1DForOutWhenUnconnected=off
  wires:
  propel_plant_init_CP_CT_map/1(output) -> propel_plant_CT_simu/1, Mux5/2
  env_plant_density_simu/1 -> Mux5/3
  propel_plant_speed_simu/1 -> propel_plant_init_CP_CT_map/1(input x), Mux5/1
  Mux5/1 -> RPS2T/1
  RPS2T/1 -> propel_plant_thrust_simu/1

== system PowerSystemRef/powerplant/propel4/plant/propel4_plant_uas/Total_Moment ==
  propel_plant_thrust_simu : Inport
  propel_plant_restq_simu : Inport  Port=2
  Gain : Gain  Gain=-propel4.plant.init.rotationdir
  Gain1 : Gain  Gain=propel4.plant.init.thrustdir
  Moment_due_to_eng_position : Subsystem
  Sum2 : Sum  Inputs=|+-  SaturateOnIntegerOverflow=on
  Sum4 : Sum  SaturateOnIntegerOverflow=on
  geom.init.CG : Constant  Value=geom.init.CG
  propel.plant.init.pos : Constant  Value=propel4.plant.init.pos
  accmoment_plant_totmoment_simu : Outport  VectorParamsAs1DForOutWhenUnconnected=off
  wires:
  propel_plant_restq_simu/1 -> Gain/1
  Gain1/1 -> Moment_due_to_eng_position/2(Vec 2)
  Gain/1 -> Sum4/2
  Sum2/1 -> Moment_due_to_eng_position/1(Vec 1)
  Sum4/1 -> accmoment_plant_totmoment_simu/1  "accmoment_plant_totmoment_simu"
  propel.plant.init.pos/1 -> Sum2/1
  geom.init.CG/1 -> Sum2/2
  propel_plant_thrust_simu/1 -> Gain1/1
  Moment_due_to_eng_position/1(X Prod) -> Sum4/1

== system PowerSystemRef/powerplant/tc/plant/tc_plant_map_trqloss_funTW/Inertia calculation ==
  inertia in : Inport
  Sum3 : Sum  Inputs=|++  InputSameDT=on  SaturateOnIntegerOverflow=on  OutDataTypeStr=Inherit: Same as first input
  tc inertia : Constant  Value=tc.plant.init.inertia
  tc.plant.init.ratio : Gain  Gain=tc.plant.init.ratio
  "tc.plant.init.ratio " : Gain  Gain=tc.plant.init.ratio
  inertia out : Outport
  wires:
  "tc.plant.init.ratio "/1 -> tc.plant.init.ratio/1
  inertia in/1 -> "tc.plant.init.ratio "/1
  tc.plant.init.ratio/1 -> Sum3/1
  tc inertia/1 -> Sum3/2
  Sum3/1 -> inertia out/1

== system PowerSystemRef/powerplant/tc/plant/tc_plant_map_trqloss_funTW/Speed calculation ==
  spd out : Inport
  tc.plant.init.ratio : Gain  Gain=tc.plant.init.ratio
  spd in : Outport
  wires:
  spd out/1 -> tc.plant.init.ratio/1
  tc.plant.init.ratio/1 -> spd in/1

== system PowerSystemRef/powerplant/tc/plant/tc_plant_map_trqloss_funTW/Torque calculation ==
  spd in : Inport
  trq in : Inport  Port=2
  Abs : Abs
  Abs1 : Abs
  Blending (state dependent) : Subsystem  mask(State dependent blending){xl=-tc.plant.init.spd_thresh, yl=-1, xc=0, yc=0, xr=tc.plant.init.spd_thresh, yr=1}
      mask prompts: xl "Left point (x):"; yl "Left point (y):"; xc "Center point (x):"; yc "Center point (y):"; xr "Right point (x):"; yr "Right point (y):"
      mask help: This block implements state dependent smoothing/blending. IMPORTANT: See help menu.
      mask Help: The output equals the product of the first input and a "hat" function defined by the three points specified in the dialog box.  The second input forms the argument to the hat function.\n\nIMPORTANT: A divide by zero error will result if first coordinates of the three points specified for the hat function are NOT distinct.
      mask Display: plot([-1 1 3 6 8], [1.5 1.5 0.5 4.0 4.0])
  Sum2 : Sum  Inputs=|+-  InputSameDT=on  SaturateOnIntegerOverflow=on  OutDataTypeStr=Inherit: Same as first input
  tc.plant.init.ratio : Gain  Gain=tc.plant.init.ratio
  trq losses : Subsystem  mask(Lookup Table (2-D)){x=tc.plant.init.trq_loss.idx1_trq, y=tc.plant.init.trq_loss.idx2_spd, t=tc.plant.init.trq_loss.map}
      mask prompts: x "Row:"; y "Column:"; t "Table:"
      mask help: Performs 2-D linear interpolation of input values using the specified input/output table. Extrapolation is performed outside the table boundaries.
      mask init:
      | [r,c]=size(t);
      | xt=reshape(x,prod(size(x)),1);
      | xi=xt(:,ones(1,c));
      | minx=min(x); maxx=max(x);
      | mint=min(min(t)); maxt=max(max(t));
      mask Display: plot(xi,t,[minx maxx],[mint mint],[minx minx],[mint maxt])
  trq out : Outport
  wires:
  tc.plant.init.ratio/1 -> trq out/1
  Sum2/1 -> tc.plant.init.ratio/1
  trq in/1 -> Sum2/1, Abs/1
  spd in/1 -> Blending (state dependent)/2(Control (state)), Abs1/1
  Blending (state dependent)/1(Output) -> Sum2/2
  trq losses/1(Out1) -> Blending (state dependent)/1(Input)
  Abs1/1 -> trq losses/2(Cols)
  Abs/1 -> trq losses/1(Rows)

== system PowerSystemRef/powerplant/tc2/plant/tc2_plant_map_trqloss_funTW/Inertia calculation ==
  inertia in : Inport
  Sum3 : Sum  Inputs=|++  InputSameDT=on  SaturateOnIntegerOverflow=on  OutDataTypeStr=Inherit: Same as first input
  tc inertia : Constant  Value=tc2.plant.init.inertia
  tc.plant.init.ratio : Gain  Gain=tc2.plant.init.ratio
  "tc.plant.init.ratio " : Gain  Gain=tc2.plant.init.ratio
  inertia out : Outport
  wires:
  "tc.plant.init.ratio "/1 -> tc.plant.init.ratio/1
  inertia in/1 -> "tc.plant.init.ratio "/1
  tc.plant.init.ratio/1 -> Sum3/1
  tc inertia/1 -> Sum3/2
  Sum3/1 -> inertia out/1

== system PowerSystemRef/powerplant/tc2/plant/tc2_plant_map_trqloss_funTW/Speed calculation ==
  spd out : Inport
  tc.plant.init.ratio : Gain  Gain=tc2.plant.init.ratio
  spd in : Outport
  wires:
  spd out/1 -> tc.plant.init.ratio/1
  tc.plant.init.ratio/1 -> spd in/1
